simulink model "simpleModelSim"  (R2021b)
settings: Solver=VariableStepAuto  StartTime=0.0  StopTime=2  RelTol=1e-3
values from neighbouring files (symbols this model uses):
  initialOmega = [droneParams.minRPM, droneParams.minRPM,                  droneParams.minRPM, droneParams.minRPM]'    [main.m]    (also in runModel.m)
  initialState = [0, 0, 0, 0, 0, 0, 0, 0, 0, 0, 0, 0]'    [main.m]    (also in runModel.m)
undefined symbols (not defined in the file or in its folder): attitude, attitude_dot, droneParams, force, modelParams, moment, omega, omega_CMD, position, position_dot, rate, rate_dot, velocity, velocity_dot
libraries: uavutilslib x1
settings Model: Creator=jbeers  LastModifiedBy=jbeers

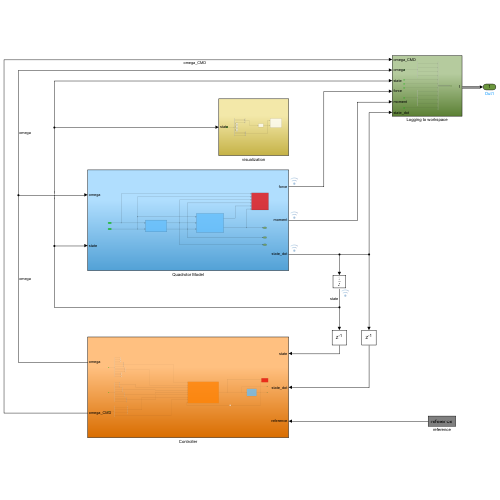
[thumbnail: Simulink's stored preview of the top-level diagram]
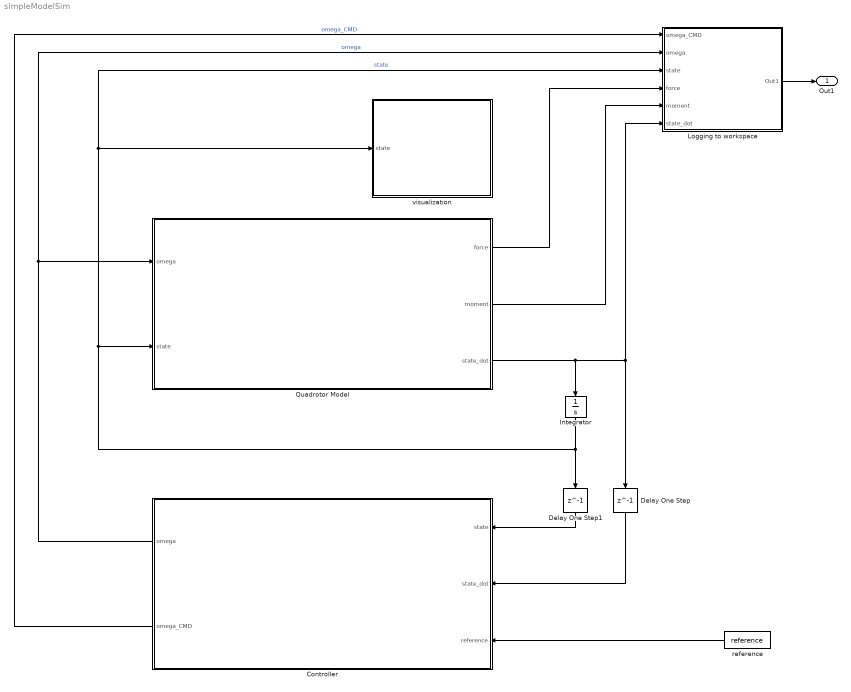
== system simpleModelSim ==
  Controller : Subsystem
  Delay One Step : Delay  DelayLength=1  InitialCondition=0
  Delay One Step1 : Delay  DelayLength=1  InitialCondition=initialState
  Integrator : Integrator
  Logging to workspace : Subsystem
  Quadrotor Model : Subsystem
  reference : FromWorkspace  VariableName=reference
  visualization : Subsystem
  Out1 : Outport
  wires:
  Quadrotor Model/3(state_dot) -> Delay One Step/1, Logging to workspace/6(state_dot), Integrator/1
  Integrator/1 -> visualization/1(state), Logging to workspace/3(state), Quadrotor Model/2(state), Delay One Step1/1  "state"
  reference/1 -> Controller/3(reference)
  Delay One Step/1 -> Controller/2(state_dot)
  Controller/1(omega) -> Quadrotor Model/1(omega), Logging to workspace/2(omega)  "omega"
  Delay One Step1/1 -> Controller/1(state)
  Logging to workspace/1(Out1) -> Out1/1
  Quadrotor Model/1(force) -> Logging to workspace/4(force)
  Quadrotor Model/2(moment) -> Logging to workspace/5(moment)
  Controller/2(omega_CMD) -> Logging to workspace/1(omega_CMD)  "omega_CMD"

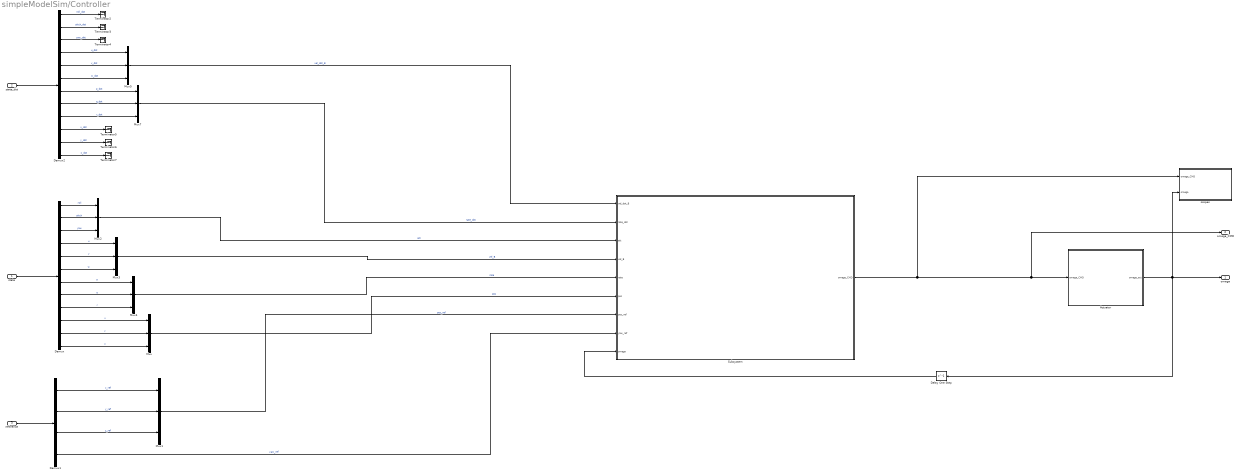
== system simpleModelSim/Controller ==
  state : Inport  PortDimensions=12
  state_dot : Inport  Port=2  PortDimensions=12
  reference : Inport  Port=3
  Actuator : Subsystem
  Delay One Step : Delay  DelayLength=1  InitialCondition=initialOmega
  Demux : Demux  Outputs=12
  Demux1 : Demux
  Demux2 : Demux  Outputs=12
  Mux{,1..5,7} (7 alike) : Mux  Inputs=3
  Subsystem : Subsystem
  Terminator{2..7} (6 alike) : Terminator
  scopes : Subsystem
  omega : Outport  PortDimensions=4
  omega_CMD : Outport  Port=2
  wires:
  state/1 -> Demux/1
  Demux/1 -> Mux2/1  "roll"
  Demux/2 -> Mux2/2  "pitch"
  Demux/3 -> Mux2/3  "yaw"
  Demux/4 -> Mux3/1  "u"
  Demux/5 -> Mux3/2  "v"
  Demux/6 -> Mux3/3  "w"
  Demux/7 -> Mux4/1  "p"
  Demux/8 -> Mux4/2  "q"
  Demux/9 -> Mux4/3  "r"
  Demux/10 -> Mux/1  "x"
  Demux/11 -> Mux/2  "y"
  Demux/12 -> Mux/3  "z"
  reference/1 -> Demux1/1
  Demux1/1 -> Mux1/1  "x_ref"
  Demux1/2 -> Mux1/2  "y_ref"
  Demux1/3 -> Mux1/3  "z_ref"
  state_dot/1 -> Demux2/1
  Demux2/1 -> Terminator2/1  "roll_dot"
  Demux2/2 -> Terminator3/1  "pitch_dot"
  Demux2/3 -> Terminator4/1  "yaw_dot"
  Demux2/4 -> Mux5/1  "u_dot"
  Demux2/5 -> Mux5/2  "v_dot"
  Demux2/6 -> Mux5/3  "w_dot"
  Demux2/7 -> Mux7/1  "p_dot"
  Demux2/8 -> Mux7/2  "q_dot"
  Demux2/9 -> Mux7/3  "r_dot"
  Demux2/10 -> Terminator5/1  "x_dot"
  Demux2/11 -> Terminator6/1  "y_dot"
  Demux2/12 -> Terminator7/1  "z_dot"
  Actuator/1(omega_act) -> omega/1, Delay One Step/1, scopes/2(omega)
  Mux5/1 -> Subsystem/1(vel_dot_B)  "vel_dot_B"
  Mux7/1 -> Subsystem/2(rate_dot)  "rate_dot"
  Mux2/1 -> Subsystem/3(att)  "att"
  Mux3/1 -> Subsystem/4(vel_B)  "vel_B"
  Mux4/1 -> Subsystem/5(rate)  "rate"
  Mux/1 -> Subsystem/6(pos)  "pos"
  Mux1/1 -> Subsystem/7(pos_ref)  "pos_ref"
  Demux1/4 -> Subsystem/8(yaw_ref)  "yaw_ref"
  Subsystem/1(omega_CMD) -> scopes/1(omega_CMD), omega_CMD/1, Actuator/1(omega_CMD)
  Delay One Step/1 -> Subsystem/9(omega)

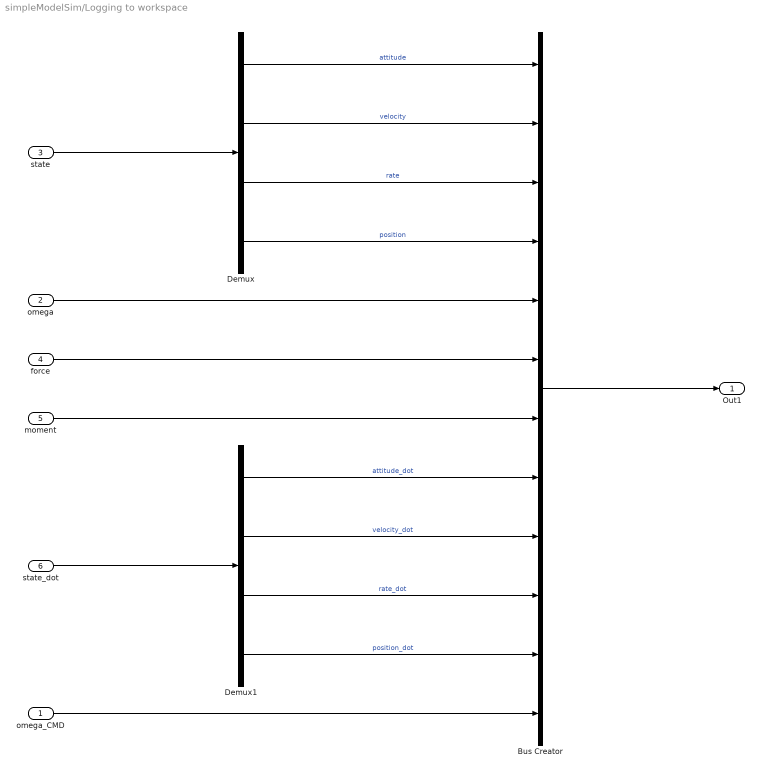
== system simpleModelSim/Logging to workspace ==
  omega_CMD : Inport
  omega : Inport  Port=2
  state : Inport  Port=3
  force : Inport  Port=4
  moment : Inport  Port=5
  state_dot : Inport  Port=6
  Bus Creator : BusCreator  Inputs=attitude,velocity,rate,position,omega,force,moment,attitude_dot,velocity_dot,rate_dot,position_dot,omega_CMD
  Demux : Demux
  Demux1 : Demux
  Out1 : Outport
  wires:
  omega/1 -> Bus Creator/5
  Bus Creator/1 -> Out1/1
  Demux/4 -> Bus Creator/4  "position"
  Demux/1 -> Bus Creator/1  "attitude"
  Demux/3 -> Bus Creator/3  "rate"
  Demux/2 -> Bus Creator/2  "velocity"
  state/1 -> Demux/1
  force/1 -> Bus Creator/6
  moment/1 -> Bus Creator/7
  Demux1/4 -> Bus Creator/11  "position_dot"
  state_dot/1 -> Demux1/1
  Demux1/2 -> Bus Creator/9  "velocity_dot"
  Demux1/1 -> Bus Creator/8  "attitude_dot"
  Demux1/3 -> Bus Creator/10  "rate_dot"
  omega_CMD/1 -> Bus Creator/12

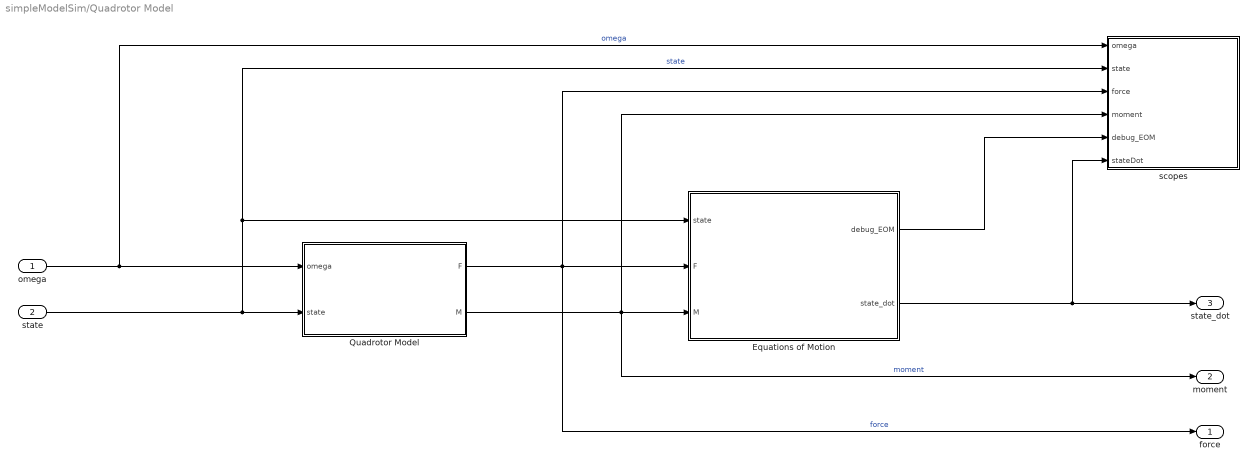
== system simpleModelSim/Quadrotor Model ==
  omega : Inport  OutMin=droneParams.minRPM  OutMax=droneParams.maxRPM  PortDimensions=4
  state : Inport  Port=2
  Equations of Motion : MATLAB Function  TreatAsAtomicUnit=on
  Quadrotor Model : MATLAB Function  TreatAsAtomicUnit=on
  scopes : Subsystem
  force : Outport
  moment : Outport  Port=2
  state_dot : Outport  Port=3
  wires:
  state/1 -> scopes/2(state), Equations of Motion/1(state), Quadrotor Model/2(state)  "state"
  Quadrotor Model/2(M) -> moment/1, scopes/4(moment), Equations of Motion/3(M)  "moment"
  Equations of Motion/2(state_dot) -> scopes/6(stateDot), state_dot/1
  omega/1 -> Quadrotor Model/1(omega), scopes/1(omega)  "omega"
  Quadrotor Model/1(F) -> force/1, Equations of Motion/2(F), scopes/3(force)  "force"
  Equations of Motion/1(debug_EOM) -> scopes/5(debug_EOM)

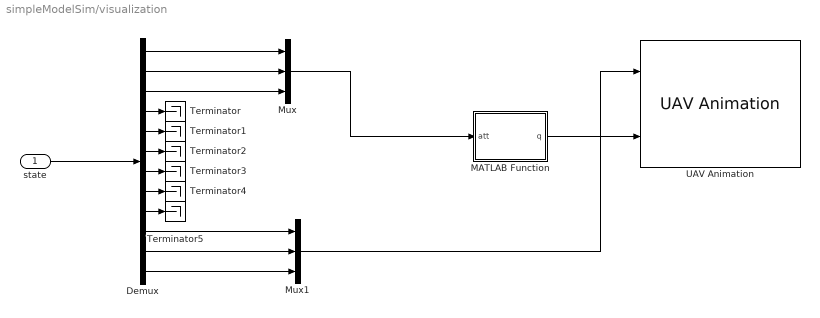
== system simpleModelSim/visualization ==
  state : Inport
  Demux : Demux  Outputs=12
  MATLAB Function : MATLAB Function  TreatAsAtomicUnit=on
  Mux : Mux  Inputs=3
  Mux1 : Mux  Inputs=3
  Terminator{,1..5} (6 alike) : Terminator
  UAV Animation : uavutilslib/UAV Animation  UAVType=Multirotor  UAVSize=2*droneParams.b  InertialZDirection=Down  SampleTime=-1
      settings: SourceProductBaseCode=UV
  wires:
  Mux1/1 -> UAV Animation/1
  Demux/3 -> Mux/3
  Demux/2 -> Mux/2
  Demux/4 -> Terminator/1
  Mux/1 -> MATLAB Function/1(att)
  Demux/11 -> Mux1/2
  Demux/12 -> Mux1/3
  Demux/1 -> Mux/1
  Demux/10 -> Mux1/1
  MATLAB Function/1(q) -> UAV Animation/2
  Demux/5 -> Terminator1/1
  state/1 -> Demux/1
  Demux/7 -> Terminator3/1
  Demux/9 -> Terminator5/1
  Demux/8 -> Terminator4/1
  Demux/6 -> Terminator2/1

== system simpleModelSim/Controller/Actuator ==
  omega_CMD : Inport
  Saturation : Saturate  UpperLimit=droneParams.maxRPM  LowerLimit=droneParams.minRPM
  omega_act : Outport
  wires:
  omega_CMD/1 -> Saturation/1
  Saturation/1 -> omega_act/1

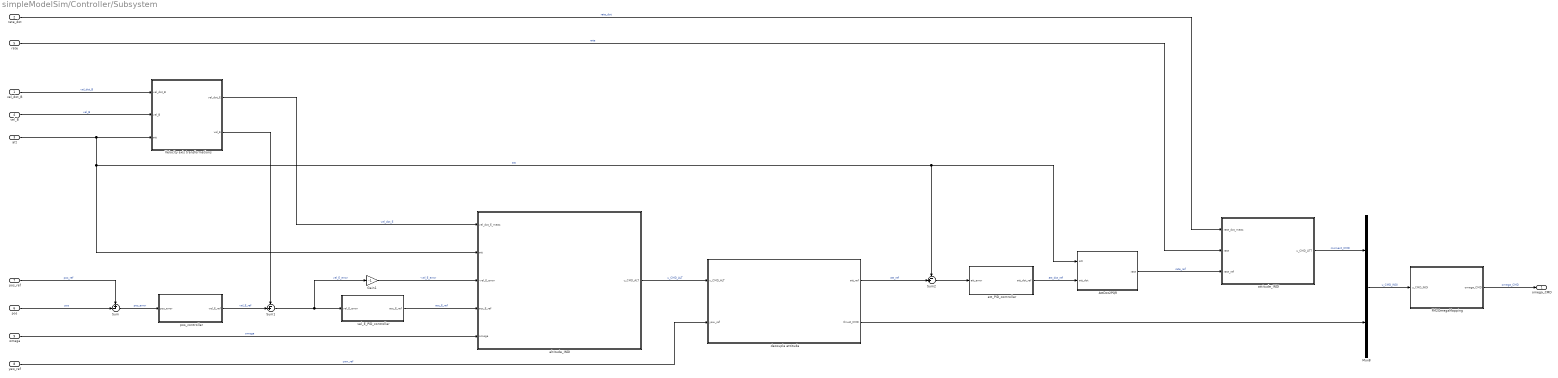
== system simpleModelSim/Controller/Subsystem ==
  vel_dot_B : Inport
  rate_dot : Inport  Port=2
  att : Inport  Port=3
  vel_B : Inport  Port=4
  rate : Inport  Port=5
  pos : Inport  Port=6
  pos_ref : Inport  Port=7
  yaw_ref : Inport  Port=8
  omega : Inport  Port=9
  AttDot2PQR : MATLAB Function  TreatAsAtomicUnit=on
  FM2OmegaMapping : MATLAB Function  TreatAsAtomicUnit=on
  Gain1 : Gain  Gain=-1
  Mux8 : Mux  Inputs=2
  Sum : Sum  Inputs=+-|
  Sum1 : Sum  Inputs=-+|
  Sum2 : Sum  Inputs=-+|
  Velocity axis transformations : Subsystem
  altitude_INDI : Subsystem
  att_PID_controller : Subsystem
  attitude_INDI : Subsystem
  decouple attitude : Subsystem
  pos_controller : Subsystem
  vel_E_PID_controller : Subsystem
  omega_CMD : Outport
  wires:
  Sum1/1 -> Gain1/1, vel_E_PID_controller/1(vel_E_error)  "vel_E_error"
  Velocity axis transformations/1(vel_dot_E) -> altitude_INDI/1(vel_dot_E_meas)  "vel_dot_E"
  rate_dot/1 -> attitude_INDI/1(rate_dot_meas)  "rate_dot"
  Sum/1 -> pos_controller/1(pos_error)  "pos_error"
  att_PID_controller/1(att_dot_ref) -> AttDot2PQR/2(att_dot)  "att_dot_ref"
  pos/1 -> Sum/2  "pos"
  omega/1 -> altitude_INDI/5(omega)  "omega"
  Mux8/1 -> FM2OmegaMapping/1(u_CMD_INDI)  "u_CMD_INDI"
  pos_ref/1 -> Sum/1  "pos_ref"
  vel_B/1 -> Velocity axis transformations/2(vel_B)  "vel_B"
  vel_E_PID_controller/1(acc_E_ref) -> altitude_INDI/4(acc_E_ref)  "acc_E_ref"
  attitude_INDI/1(u_CMD_ATT) -> Mux8/1  "moment_CMD"
  Velocity axis transformations/2(vel_E) -> Sum1/1
  yaw_ref/1 -> decouple attitude/2(yaw_ref)  "yaw_ref"
  att/1 -> altitude_INDI/2(att), Sum2/1, AttDot2PQR/1(att), Velocity axis transformations/3(att)  "att"
  Gain1/1 -> altitude_INDI/3(-vel_E_error)  "-vel_E_error"
  altitude_INDI/1(u_CMD_ALT) -> decouple attitude/1(u_CMD_ALT)  "u_CMD_ALT"
  decouple attitude/1(att_ref) -> Sum2/2  "att_ref"
  FM2OmegaMapping/1(omega_CMD) -> omega_CMD/1  "omega_CMD"
  Sum2/1 -> att_PID_controller/1(att_error)
  rate/1 -> attitude_INDI/2(rate)  "rate"
  pos_controller/1(vel_E_ref) -> Sum1/2  "vel_E_ref"
  vel_dot_B/1 -> Velocity axis transformations/1(vel_dot_B)  "vel_dot_B"
  decouple attitude/2(thrust_CMD) -> Mux8/2
  AttDot2PQR/1(rate) -> attitude_INDI/3(rate_ref)  "rate_ref"

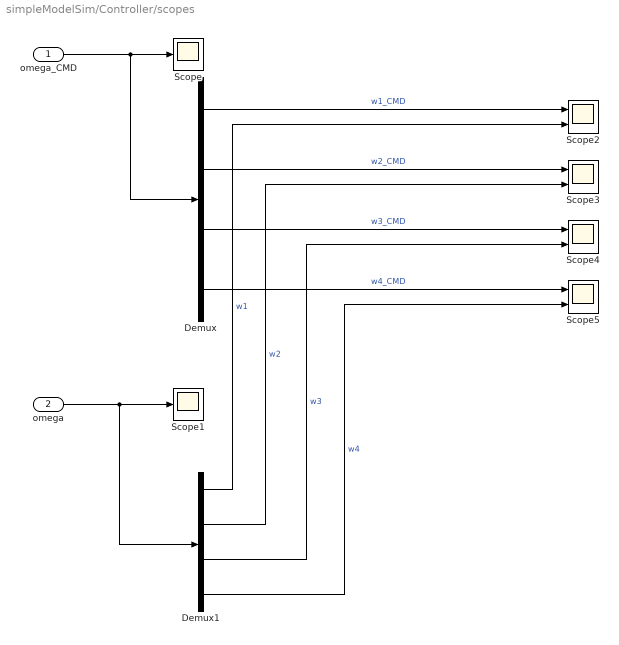
== system simpleModelSim/Controller/scopes ==
  omega_CMD : Inport
  omega : Inport  Port=2
  Demux : Demux
  Demux1 : Demux
  Scope : Scope
  Scope1 : Scope
  Scope{2..5} (4 alike) : Scope  NumInputPorts=2
  wires:
  omega_CMD/1 -> Demux/1, Scope/1
  omega/1 -> Demux1/1, Scope1/1
  Demux/1 -> Scope2/1  "w1_CMD"
  Demux1/1 -> Scope2/2  "w1"
  Demux/2 -> Scope3/1  "w2_CMD"
  Demux1/2 -> Scope3/2  "w2"
  Demux/3 -> Scope4/1  "w3_CMD"
  Demux1/3 -> Scope4/2  "w3"
  Demux/4 -> Scope5/1  "w4_CMD"
  Demux1/4 -> Scope5/2  "w4"

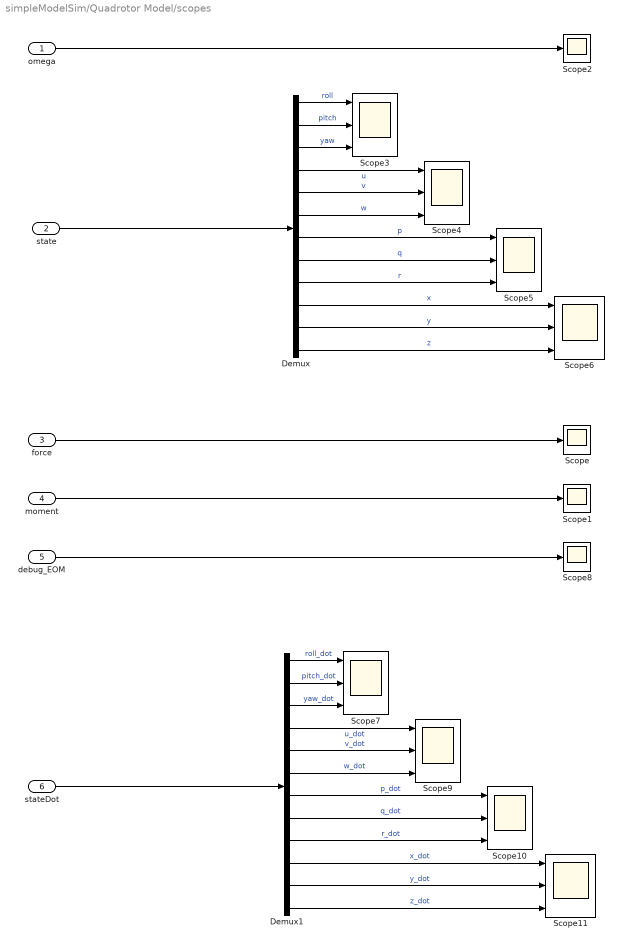
== system simpleModelSim/Quadrotor Model/scopes ==
  omega : Inport
  state : Inport  Port=2
  force : Inport  Port=3
  moment : Inport  Port=4
  debug_EOM : Inport  Port=5
  stateDot : Inport  Port=6
  Demux : Demux  Outputs=12
  Demux1 : Demux  Outputs=12
  Scope{,1..2,8} (4 alike) : Scope
  Scope{3..7,9..11} (8 alike) : Scope  NumInputPorts=3
  wires:
  Demux/12 -> Scope6/3  "z"
  Demux/7 -> Scope5/1  "p"
  Demux/8 -> Scope5/2  "q"
  Demux/1 -> Scope3/1  "roll"
  Demux/2 -> Scope3/2  "pitch"
  Demux/5 -> Scope4/2  "v"
  Demux/11 -> Scope6/2  "y"
  Demux/10 -> Scope6/1  "x"
  Demux/3 -> Scope3/3  "yaw"
  omega/1 -> Scope2/1
  Demux/9 -> Scope5/3  "r"
  Demux/4 -> Scope4/1  "u"
  Demux/6 -> Scope4/3  "w"
  state/1 -> Demux/1
  debug_EOM/1 -> Scope8/1
  force/1 -> Scope/1
  moment/1 -> Scope1/1
  Demux1/3 -> Scope7/3  "yaw_dot"
  stateDot/1 -> Demux1/1
  Demux1/6 -> Scope9/3  "w_dot"
  Demux1/4 -> Scope9/1  "u_dot"
  Demux1/9 -> Scope10/3  "r_dot"
  Demux1/10 -> Scope11/1  "x_dot"
  Demux1/5 -> Scope9/2  "v_dot"
  Demux1/2 -> Scope7/2  "pitch_dot"
  Demux1/11 -> Scope11/2  "y_dot"
  Demux1/1 -> Scope7/1  "roll_dot"
  Demux1/12 -> Scope11/3  "z_dot"
  Demux1/8 -> Scope10/2  "q_dot"
  Demux1/7 -> Scope10/1  "p_dot"

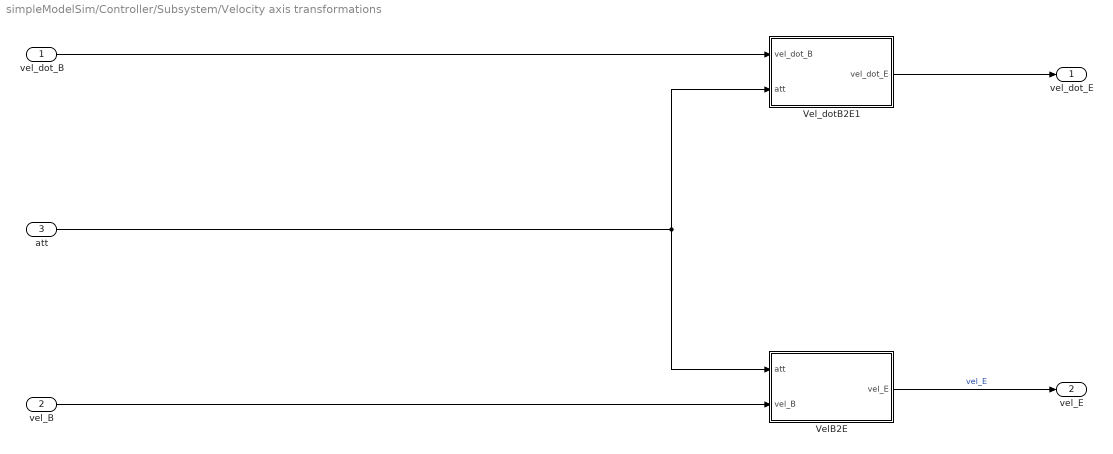
== system simpleModelSim/Controller/Subsystem/Velocity axis transformations ==
  vel_dot_B : Inport
  vel_B : Inport  Port=2
  att : Inport  Port=3
  VelB2E : MATLAB Function  TreatAsAtomicUnit=on
  Vel_dotB2E1 : MATLAB Function  TreatAsAtomicUnit=on
  vel_dot_E : Outport
  vel_E : Outport  Port=2
  wires:
  att/1 -> VelB2E/1(att), Vel_dotB2E1/2(att)
  VelB2E/1(vel_E) -> vel_E/1  "vel_E"
  Vel_dotB2E1/1(vel_dot_E) -> vel_dot_E/1
  vel_dot_B/1 -> Vel_dotB2E1/1(vel_dot_B)
  vel_B/1 -> VelB2E/2(vel_B)

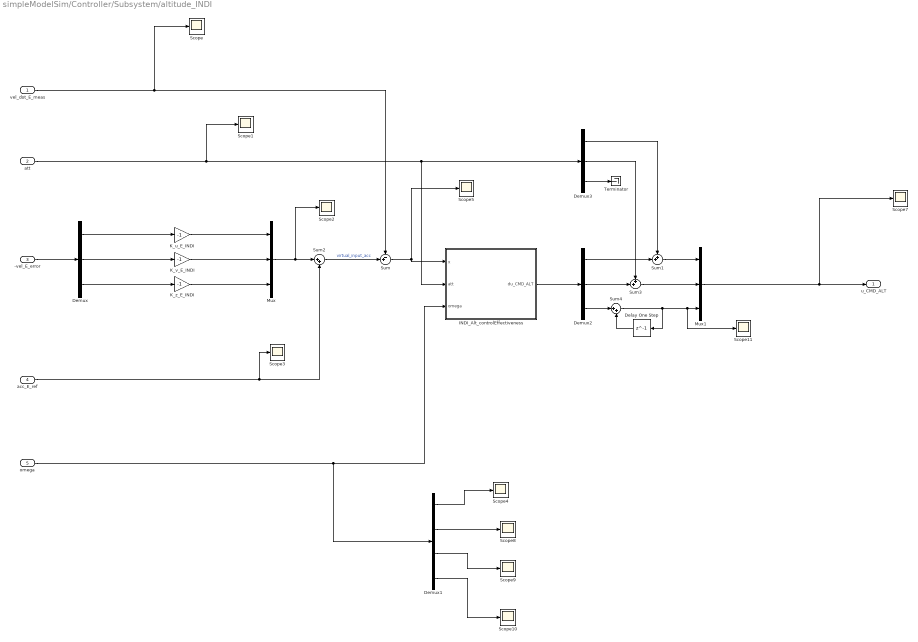
== system simpleModelSim/Controller/Subsystem/altitude_INDI ==
  vel_dot_E_meas : Inport
  att : Inport  Port=2
  -vel_E_error : Inport  Port=3
  acc_E_ref : Inport  Port=4
  omega : Inport  Port=5
  Delay One Step : Delay  DelayLength=1
  Demux : Demux  Outputs=3
  Demux1 : Demux
  Demux2 : Demux  Outputs=3
  Demux3 : Demux  Outputs=3
  INDI_Alt_controlEffectiveness : MATLAB Function  TreatAsAtomicUnit=on
  K_u_E_INDI : Gain  Gain=-1
  K_v_E_INDI : Gain  Gain=-1
  K_z_E_INDI : Gain  Gain=-1
  Mux : Mux  Inputs=3
  Mux1 : Mux  Inputs=3
  Scope{,1..5,7..11} (11 alike) : Scope
  Sum : Sum  Inputs=-+|
  Sum1 : Sum  Inputs=++|
  Sum2 : Sum  Inputs=|++
  Sum3 : Sum  Inputs=++|
  Sum4 : Sum  Inputs=|++
  Terminator : Terminator
  u_CMD_ALT : Outport
  wires:
  K_v_E_INDI/1 -> Mux/2
  K_z_E_INDI/1 -> Mux/3
  Demux/3 -> K_z_E_INDI/1
  Demux/2 -> K_v_E_INDI/1
  Demux/1 -> K_u_E_INDI/1
  -vel_E_error/1 -> Demux/1
  K_u_E_INDI/1 -> Mux/1
  Mux/1 -> Scope2/1, Sum2/1
  acc_E_ref/1 -> Scope3/1, Sum2/2
  Sum2/1 -> Sum/2  "virtual_input_acc"
  vel_dot_E_meas/1 -> Scope/1, Sum/1
  Sum/1 -> INDI_Alt_controlEffectiveness/1(x), Scope5/1
  omega/1 -> INDI_Alt_controlEffectiveness/3(omega), Demux1/1
  INDI_Alt_controlEffectiveness/1(du_CMD_ALT) -> Demux2/1
  Mux1/1 -> Scope7/1, u_CMD_ALT/1
  Demux1/1 -> Scope4/1
  Demux1/2 -> Scope8/1
  Demux1/3 -> Scope9/1
  Demux1/4 -> Scope10/1
  Demux2/1 -> Sum1/2
  Demux3/1 -> Sum1/1
  Demux3/3 -> Terminator/1
  Demux3/2 -> Sum3/1
  Demux2/2 -> Sum3/2
  Sum3/1 -> Mux1/2
  Sum1/1 -> Mux1/1
  Demux2/3 -> Sum4/1
  Sum4/1 -> Delay One Step/1, Scope11/1, Mux1/3
  att/1 -> Scope1/1, Demux3/1, INDI_Alt_controlEffectiveness/2(att)
  Delay One Step/1 -> Sum4/2

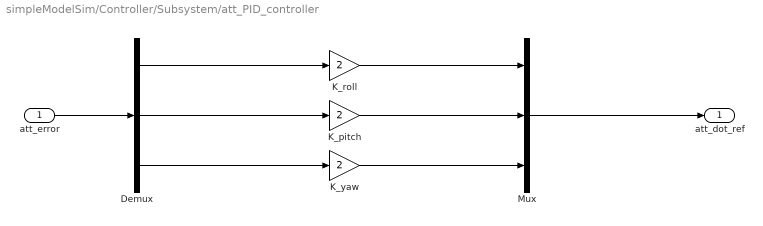
== system simpleModelSim/Controller/Subsystem/att_PID_controller ==
  att_error : Inport
  Demux : Demux  Outputs=3
  K_pitch : Gain  Gain=2
  K_roll : Gain  Gain=2
  K_yaw : Gain  Gain=2
  Mux : Mux  Inputs=3
  att_dot_ref : Outport
  wires:
  att_error/1 -> Demux/1
  Demux/1 -> K_roll/1
  Demux/2 -> K_pitch/1
  Demux/3 -> K_yaw/1
  K_roll/1 -> Mux/1
  K_pitch/1 -> Mux/2
  K_yaw/1 -> Mux/3
  Mux/1 -> att_dot_ref/1

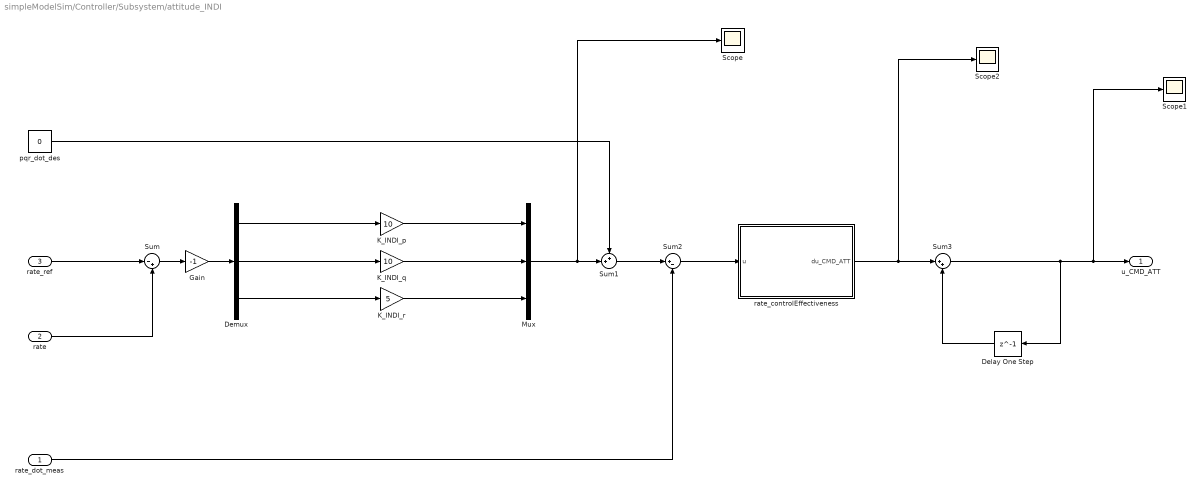
== system simpleModelSim/Controller/Subsystem/attitude_INDI ==
  rate_dot_meas : Inport
  rate : Inport  Port=2
  rate_ref : Inport  Port=3
  Delay One Step : Delay  DelayLength=1
  Demux : Demux  Outputs=3
  Gain : Gain  Gain=-1
  K_INDI_p : Gain  Gain=10
  K_INDI_q : Gain  Gain=10
  K_INDI_r : Gain  Gain=5
  Mux : Mux  Inputs=3
  Scope : Scope
  Scope1 : Scope
  Scope2 : Scope
  Sum : Sum  Inputs=|-+
  Sum1 : Sum  Inputs=++|
  Sum2 : Sum  Inputs=|+-
  Sum3 : Sum  Inputs=|++
  pqr_dot_des : Constant  Value=0
  rate_controlEffectiveness : MATLAB Function  TreatAsAtomicUnit=on
  u_CMD_ATT : Outport
  wires:
  Demux/1 -> K_INDI_p/1
  Sum/1 -> Gain/1
  Mux/1 -> Scope/1, Sum1/2
  K_INDI_r/1 -> Mux/3
  K_INDI_q/1 -> Mux/2
  K_INDI_p/1 -> Mux/1
  Demux/2 -> K_INDI_q/1
  Demux/3 -> K_INDI_r/1
  rate_ref/1 -> Sum/1
  rate/1 -> Sum/2
  pqr_dot_des/1 -> Sum1/1
  rate_dot_meas/1 -> Sum2/2
  Sum1/1 -> Sum2/1
  Sum2/1 -> rate_controlEffectiveness/1(u)
  rate_controlEffectiveness/1(du_CMD_ATT) -> Scope2/1, Sum3/1
  Sum3/1 -> Scope1/1, u_CMD_ATT/1, Delay One Step/1
  Delay One Step/1 -> Sum3/2
  Gain/1 -> Demux/1

== system simpleModelSim/Controller/Subsystem/decouple attitude ==
  u_CMD_ALT : Inport
  yaw_ref : Inport  Port=2
  Demux4 : Demux  Outputs=3
  Gain : Gain  Gain=-1
  Mux6 : Mux  Inputs=3
  att_ref : Outport
  thrust_CMD : Outport  Port=2
  wires:
  Demux4/1 -> Mux6/1  "roll_ref"
  Demux4/3 -> thrust_CMD/1  "thrust_CMD"
  yaw_ref/1 -> Mux6/3
  Demux4/2 -> Mux6/2  "pitch_ref"
  Gain/1 -> Demux4/1
  Mux6/1 -> att_ref/1  "att_ref"
  u_CMD_ALT/1 -> Gain/1

== system simpleModelSim/Controller/Subsystem/pos_controller ==
  pos_error : Inport
  Demux : Demux  Outputs=3
  K_x : Gain
  K_y : Gain
  K_z : Gain  Gain=1.5
  Mux : Mux  Inputs=3
  vel_E_ref : Outport
  wires:
  pos_error/1 -> Demux/1
  Demux/1 -> K_x/1
  Demux/2 -> K_y/1
  Demux/3 -> K_z/1
  K_x/1 -> Mux/1
  K_y/1 -> Mux/2
  K_z/1 -> Mux/3
  Mux/1 -> vel_E_ref/1

== system simpleModelSim/Controller/Subsystem/vel_E_PID_controller ==
  vel_E_error : Inport
  Demux : Demux  Outputs=3
  K_u_E : Gain  Gain=2.5
  K_v_E : Gain  Gain=2.5
  K_w_E : Gain  Gain=3
  Mux : Mux  Inputs=3
  acc_E_ref : Outport
  wires:
  K_u_E/1 -> Mux/1
  Demux/1 -> K_u_E/1
  Demux/3 -> K_w_E/1
  K_w_E/1 -> Mux/3
  K_v_E/1 -> Mux/2
  vel_E_error/1 -> Demux/1
  Demux/2 -> K_v_E/1
  Mux/1 -> acc_E_ref/1

== matlab function simpleModelSim/Quadrotor Model/Equations of Motion ==
  data: debug_EOM output; state input; F input; state_dot output; M input; droneParams parameter; modelParams parameter
% function state_dot = EOM(state, F, M, droneParams, modelParams)
function [debug_EOM, state_dot] = EOM(state, F, M, droneParams, modelParams)
    % Function to compute the quadrotor equations of motion
    % state = [roll, pitch, yaw, u, v, w, p, q, r, x, y, z]
    %   - Attitude: [roll, pitch, yaw] in rad
    %   - (Body) velocity: [u, v, w] in m/s
    %   - (Body) rotational rates: [p, q, r] in rad/s
    %   - Position: [x, y, z] in E-frame, in m

    % Extract necessary drone parameters
    mass = droneParams.mass;
    Iv = droneParams.Iv;
    invIv = inv(Iv);
    g = modelParams.g;
    gVec = [0; 0; g];

    % Pre-allocate state derivative array
    state_dot = zeros(size(state));

    % Compute accelerations
    linAcc = (F/mass)' + QuatRot(gVec, state(1:3), "E2B") - cross(state(7:9), state(4:6));
    rotAcc = invIv*M' - invIv * (cross(state(7:9), Iv*state(7:9)));

    % Fill in state derivative
    state_dot(1:3) = PQR_to_AttDot_Euler(state(1:3), state(7:9));
    state_dot(4:6) = linAcc;
    state_dot(7:9) = rotAcc;
    state_dot(10:12) = QuatRot(state(4:6), state(1:3), "B2E");

    % Debugging
    debug_EOM = 0;

== matlab function simpleModelSim/Quadrotor Model/Quadrotor Model ==
  data: omega input; state input; F output; M output; droneParams parameter; modelParams parameter
function [F, M] = getForcesMoments(omega, state, droneParams, modelParams)
    % Call function getFM() from workspace
    [F, M] = getFM(state, omega, modelParams, droneParams);

== matlab function simpleModelSim/Controller/Subsystem/Velocity axis transformations/VelB2E ==
  data: att input; vel_B input; vel_E output
function vel_E = VelB2E(att, vel_B)
    % Rotate velocity from body frame to earth frame
    vel_E = QuatRot(vel_B, att, "B2E");

== matlab function simpleModelSim/Controller/Subsystem/Velocity axis transformations/Vel_dotB2E1 ==
  data: vel_dot_B input; att input; vel_dot_E output
function vel_dot_E = VelB2E(vel_dot_B, att)
    % Rotate velocity from body frame to earth frame
    vel_dot_E = QuatRot(vel_dot_B, att, "B2E");

== matlab function simpleModelSim/Controller/Subsystem/altitude_INDI/INDI_Alt_controlEffectiveness ==
  data: x input; att input; du_CMD_ALT output; omega input; droneParams parameter
function du_CMD_ALT  = INDI_ALT_B(x, att, omega, droneParams)
    cPhi = cos(att(1));
    sPhi = sin(att(1));
    cTheta = cos(att(2));
    sTheta = sin(att(2));
    cPsi = cos(att(3));
    sPsi = sin(att(3));    

    T = sum(droneParams.kappaFz .* (omega.^2));

    G = [
        [(cPhi*sPsi - sPhi*cPsi*sTheta)*T, (cPhi*cPsi*cTheta)*T, sPhi*sPsi + cPhi*cPsi*sTheta];
        [(-1*sPhi*sPsi*sTheta - cPsi*cPhi)*T, (cPhi*sPsi*cTheta)*T, cPhi*sPsi*sTheta - cPsi*sPhi];
        [(-cTheta*sPhi)*T, -sTheta*cPhi*T, cPhi*cTheta]
    ];
    
    du_CMD_ALT = droneParams.mass * (G \ x);

== matlab function simpleModelSim/Controller/Subsystem/AttDot2PQR ==
  data: att input; rate output; att_dot input
function rate  = AttDot2PQR(att, att_dot)
    [rate] = AttDot_to_PQR_Euler(att, att_dot);

== matlab function simpleModelSim/Controller/Subsystem/attitude_INDI/rate_controlEffectiveness ==
  data: u input; du_CMD_ATT output; droneParams parameter
function du_CMD_ATT = controllEffectiveness_ATT(u, droneParams)
    du_CMD_ATT = droneParams.Iv*u;

== matlab function simpleModelSim/Controller/Subsystem/FM2OmegaMapping ==
  data: u_CMD_INDI input; omega_CMD output; droneParams parameter
function omega_CMD  = FM2OmegaMapping(u_CMD_INDI, droneParams)
    Mapping = droneParams.FM2OmegaMapping;
    
    u2 = Mapping*u_CMD_INDI;

    u2(u2 < 0) = 0;

    omega_CMD = sqrt(u2);

== matlab function simpleModelSim/visualization/MATLAB Function ==
  data: att input; q output
function q = E2Q(att)

q = Eul2Quat(att);
